simulink model "ADRC_test"  (R2015a)
settings: Solver=ode3  SolverMode=SingleTasking  StartTime=0.0  StopTime=100  RelTol=1e-3
undefined symbols (not defined in the file or in its folder): alpha1, alpha2, b, beta01, beta02, beta03, delta, h, h0, nlsef_alpha1, nlsef_alpha2, r
settings Model: CovMetricSettings=dwe  CovHtmlReporting=off  covSaveCumulativeToWorkspaceVar=off  CovSaveSingleToWorkspaceVar=off  CovExternalEMLEnable=on  Creator=c  LastModifiedBy=DELL
settings DataIOCC: LimitDataPoints=off  SaveFormat=Dataset  ReturnWorkspaceOutputs=on
settings DebuggingCC: SFUnexpectedBacktrackingDiag=error  SFNoUnconditionalDefaultTransitionDiag=error
settings HardwareCC: ProdBitPerPointer=64  ProdLargestAtomicFloat=Float  ProdIntDivRoundTo=Zero  ProdEndianess=LittleEndian  ProdHWDeviceType=Specified
settings ModelReferenceCC: PropagateSignalLabelsOutOfModel=on
settings SFSimCC: SimUseLocalCustomCode=on
settings RTWCC: RTWUseLocalCustomCode=on
settings GRTTargetCC: TargetLangStandard=C99 (ISO)

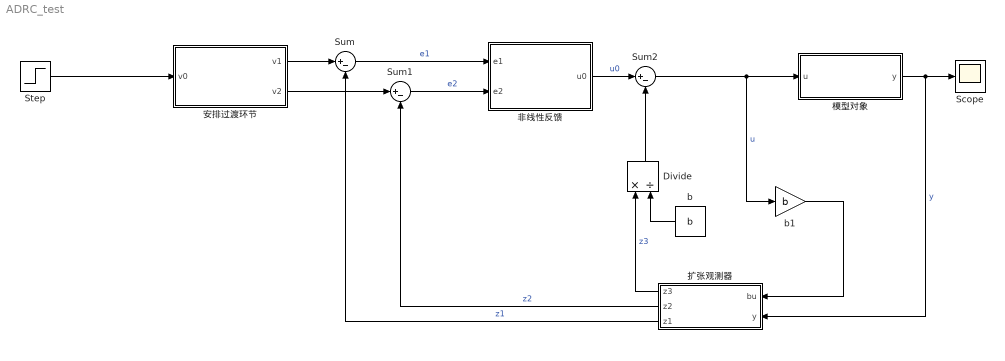
== system ADRC_test ==
  Divide : Product  Inputs=*/
  Scope : Scope
      settings: TimeRange=auto  MaxDataPoints=5000  SaveToWorkspace=off  SaveName=ScopeData  YMin=-0.125  YMax=1.125  SampleTime=-1
  Step : Step  Time=20  SampleTime=0.01
  Sum : Sum  Inputs=|+-
  Sum1 : Sum  Inputs=|+-
  Sum2 : Sum  Inputs=|+-
  b : Constant  Value=b
  b1 : Gain  Gain=b
  安排过渡环节 : Subsystem
  扩张观测器 : Subsystem
  模型对象 : Subsystem
  非线性反馈 : Subsystem
  wires:
  安排过渡环节/1(v1) -> Sum/1
  安排过渡环节/2(v2) -> Sum1/1
  扩张观测器/3(z1) -> Sum/2  "z1"
  扩张观测器/2(z2) -> Sum1/2  "z2"
  Sum/1 -> 非线性反馈/1(e1)  "e1"
  Sum1/1 -> 非线性反馈/2(e2)  "e2"
  Sum2/1 -> b1/1, 模型对象/1(u)  "u"
  非线性反馈/1(u0) -> Sum2/1  "u0"
  Divide/1 -> Sum2/2
  b/1 -> Divide/2
  扩张观测器/1(z3) -> Divide/1  "z3"
  模型对象/1(y) -> 扩张观测器/2(y), Scope/1  "y"
  b1/1 -> 扩张观测器/1(bu)
  Step/1 -> 安排过渡环节/1(v0)

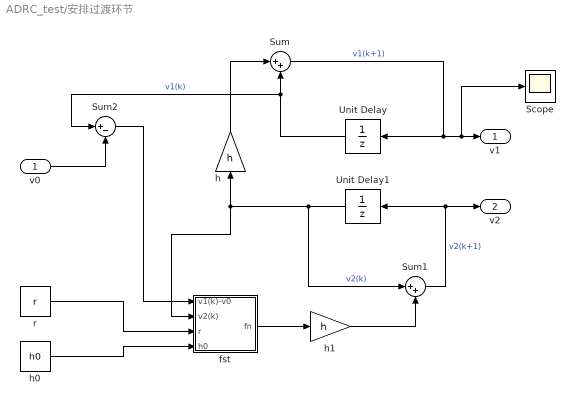
== system ADRC_test/安排过渡环节 ==
  v0 : Inport
  Scope : Scope
      settings: TimeRange=auto  MaxDataPoints=5000  SaveToWorkspace=off  YMin=-0.125  YMax=1.125  SampleTime=-1
  Sum : Sum  Inputs=|++
  Sum1 : Sum  Inputs=|++
  Sum2 : Sum  Inputs=|+-
  Unit Delay : UnitDelay  SampleTime=-1  HasFrameUpgradeWarning=on
  Unit Delay1 : UnitDelay  SampleTime=-1  HasFrameUpgradeWarning=on
  fst : Subsystem
  h : Gain  Gain=h
  h0 : Constant  Value=h0
  h1 : Gain  Gain=h
  r : Constant  Value=r
  v1 : Outport
  v2 : Outport  Port=2
  wires:
  Sum1/1 -> Unit Delay1/1, v2/1  "v2(k+1)"
  Sum/1 -> Unit Delay/1, Scope/1, v1/1  "v1(k+1)"
  Unit Delay/1 -> Sum2/1, Sum/2  "v1(k)"
  Unit Delay1/1 -> Sum1/1, fst/2(v2(k)), h/1  "v2(k)"
  h/1 -> Sum/1
  fst/1(fn) -> h1/1
  h1/1 -> Sum1/2
  r/1 -> fst/3(r)
  h0/1 -> fst/4(h0)
  v0/1 -> Sum2/2
  Sum2/1 -> fst/1(v1(k)-v0)

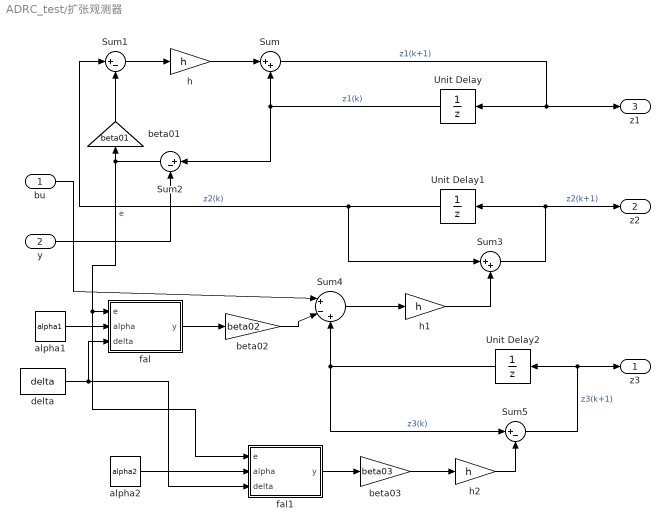
== system ADRC_test/扩张观测器 ==
  bu : Inport
  y : Inport  Port=2
  Sum : Sum  Inputs=|++
  Sum1 : Sum  Inputs=|+-
  Sum2 : Sum  Inputs=|+-
  Sum3 : Sum  Inputs=|++
  Sum4 : Sum  Inputs=|+-+
  Sum5 : Sum  Inputs=|+-
  Unit Delay : UnitDelay  SampleTime=-1  HasFrameUpgradeWarning=on
  Unit Delay1 : UnitDelay  SampleTime=-1  HasFrameUpgradeWarning=on
  Unit Delay2 : UnitDelay  SampleTime=-1  HasFrameUpgradeWarning=on
  alpha1 : Constant  Value=alpha1
  alpha2 : Constant  Value=alpha2
  beta01 : Gain  Gain=beta01
  beta02 : Gain  Gain=beta02
  beta03 : Gain  Gain=beta03
  delta : Constant  Value=delta
  fal : MATLAB Function  TreatAsAtomicUnit=on
      settings: PermitHierarchicalResolution=ParametersOnly
  fal1 : MATLAB Function  TreatAsAtomicUnit=on
      settings: PermitHierarchicalResolution=ParametersOnly
  h : Gain  Gain=h
  h1 : Gain  Gain=h
  h2 : Gain  Gain=h
  z3 : Outport
  z2 : Outport  Port=2
  z1 : Outport  Port=3
  wires:
  Sum/1 -> Unit Delay/1, z1/1  "z1(k+1)"
  Unit Delay/1 -> Sum2/1, Sum/2  "z1(k)"
  Sum3/1 -> Unit Delay1/1, z2/1  "z2(k+1)"
  Unit Delay1/1 -> Sum3/1, Sum1/1  "z2(k)"
  h/1 -> Sum/1
  beta01/1 -> Sum1/2
  Sum2/1 -> fal1/1(e), fal/1(e), beta01/1  "e"
  y/1 -> Sum2/2
  Sum1/1 -> h/1
  h1/1 -> Sum3/2
  Sum4/1 -> h1/1
  Sum5/1 -> z3/1, Unit Delay2/1  "z3(k+1)"
  Unit Delay2/1 -> Sum5/1, Sum4/3  "z3(k)"
  beta02/1 -> Sum4/2
  fal/1(y) -> beta02/1
  bu/1 -> Sum4/1
  alpha1/1 -> fal/2(alpha)
  delta/1 -> fal1/3(delta), fal/3(delta)
  h2/1 -> Sum5/2
  beta03/1 -> h2/1
  fal1/1(y) -> beta03/1
  alpha2/1 -> fal1/2(alpha)

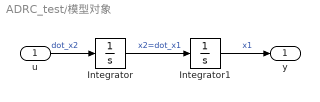
== system ADRC_test/模型对象 ==
  u : Inport
  Integrator : Integrator
  Integrator1 : Integrator  InitialCondition=0.5
  y : Outport
  wires:
  u/1 -> Integrator/1  "dot_x2"
  Integrator/1 -> Integrator1/1  "x2=dot_x1"
  Integrator1/1 -> y/1  "x1"

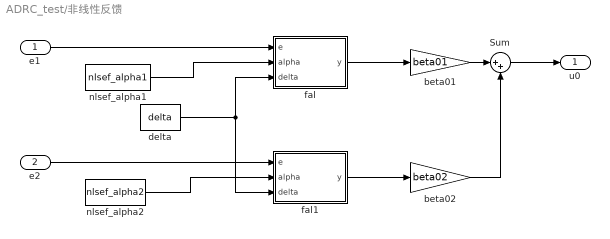
== system ADRC_test/非线性反馈 ==
  e1 : Inport
  e2 : Inport  Port=2
  Sum : Sum  Inputs=|++
  beta01 : Gain  Gain=beta01
  beta02 : Gain  Gain=beta02
  delta : Constant  Value=delta
  fal : MATLAB Function  TreatAsAtomicUnit=on
      settings: PermitHierarchicalResolution=ParametersOnly
  fal1 : MATLAB Function  TreatAsAtomicUnit=on
      settings: PermitHierarchicalResolution=ParametersOnly
  nlsef_alpha1 : Constant  Value=nlsef_alpha1
  nlsef_alpha2 : Constant  Value=nlsef_alpha2
  u0 : Outport
  wires:
  e1/1 -> fal/1(e)
  nlsef_alpha1/1 -> fal/2(alpha)
  e2/1 -> fal1/1(e)
  nlsef_alpha2/1 -> fal1/2(alpha)
  delta/1 -> fal1/3(delta), fal/3(delta)
  fal/1(y) -> beta01/1
  fal1/1(y) -> beta02/1
  beta01/1 -> Sum/1
  beta02/1 -> Sum/2
  Sum/1 -> u0/1

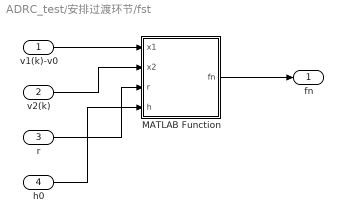
== system ADRC_test/安排过渡环节/fst ==
  v1(k)-v0 : Inport
  v2(k) : Inport  Port=2
  r : Inport  Port=3
  h0 : Inport  Port=4
  MATLAB Function : MATLAB Function  TreatAsAtomicUnit=on
      settings: PermitHierarchicalResolution=ParametersOnly
  fn : Outport
  wires:
  v1(k)-v0/1 -> MATLAB Function/1(x1)
  v2(k)/1 -> MATLAB Function/2(x2)
  r/1 -> MATLAB Function/3(r)
  h0/1 -> MATLAB Function/4(h)
  MATLAB Function/1(fn) -> fn/1

== matlab function ADRC_test/非线性反馈/fal ==
  data: e input; y output; alpha input; delta input
%fal函数
function y=fal(e,alpha,delta)
    if abs(e)>delta
        y=abs(e)^alpha*sign(e);
    else
        y=e/(delta^(1-alpha));
    end
end

== matlab function ADRC_test/安排过渡环节/fst/MATLAB Function ==
  data: x1 input; fn output; x2 input; r input; h input
%fst函数
function fn=fst(x1,x2,r,h)
    d=h*r;
    d0=h*d;
    y=x1+h*x2;
    a0=sqrt(d^2+8*r*abs(y));

    if abs(y)<=d0
        a=x2+y/h;
    else
        a=x2+0.5*(a0-d)*sgn(y);
    end
    fn=-r*sat(a,d);
end

== matlab function ADRC_test/非线性反馈/fal1 ==
  data: e input; y output; alpha input; delta input
%fal函数
function y=fal(e,alpha,delta)
    if abs(e)>delta
        y=abs(e)^alpha*sign(e);
    else
        y=e/(delta^(1-alpha));
    end
end

== matlab function ADRC_test/扩张观测器/fal ==
  data: e input; y output; alpha input; delta input
%fal函数
function y=fal(e,alpha,delta)
    if abs(e)>delta
        y=abs(e)^alpha*sign(e);
    else
        y=e/(delta^(1-alpha));
    end
end

== matlab function ADRC_test/扩张观测器/fal1 ==
  data: e input; y output; alpha input; delta input
%fal函数
function y=fal(e,alpha,delta)
    if abs(e)>delta
        y=abs(e)^alpha*sign(e);
    else
        y=e/(delta^(1-alpha));
    end
end
